simulink model "gm_interleaver_model"  (R2020b)
settings: Solver=FixedStepDiscrete  StartTime=0.0  StopTime=30  RelTol=1e-3
libraries: commrandsrc3 x1, hdlsllib x1
settings Model: Creator=wardo  LastModifiedBy=EFlores
settings DataIOCC: LimitDataPoints=on  SaveOutput=off  SaveTime=off
settings OptimizationCC: BlockReduction=off  ConditionallyExecuteInputs=off  DefaultParameterBehavior=Inlined  LifeSpan=inf
settings DebuggingCC: AlgebraicLoopMsg=error  InheritedTsInSrcMsg=none  SingleTaskRateTransMsg=error  AllowSymbolicDim=off  StrictBusMsg=ErrorOnBusTreatedAsVector  SFUnexpectedBacktrackingDiag=warning  SFNoUnconditionalDefaultTransitionDiag=warning  SFExecutionAtInitializationDiag=none  ArithmeticOperatorsInVariantConditions=warning
settings HardwareCC: ProdBitPerPointer=32  ProdBitPerSizeT=32  ProdBitPerPtrDiffT=32  ProdLargestAtomicFloat=None  ProdIntDivRoundTo=Undefined  ProdEndianess=Unspecified  ProdWordSize=32  ProdHWDeviceType=ASIC/FPGA->ASIC/FPGA  ProdEqTarget=off
settings SFSimCC: SimUseLocalCustomCode=off  CustomCodeUndefinedFunction=UseInterfaceOnly
settings RTWCC: RTWUseLocalCustomCode=off
settings CodeAppCC: StateflowObjectComments=on
settings GRTTargetCC: TargetLangStandard=C89/C90 (ANSI)
settings ConfigComp: CovScope=ReferencedModels  CovMetricSettings=dw  CovSaveCumulativeToWorkspaceVar=on  CovSaveSingleToWorkspaceVar=on  CovExternalEMLEnable=off  CovSFcnEnable=off

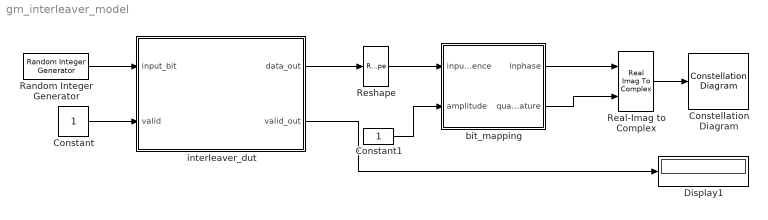
== system gm_interleaver_model ==
  Constant : Constant  OutDataTypeStr=boolean  SampleTime=-1
  Constant1 : Constant  OutMin=0  OutMax=5  OutDataTypeStr=fixdt(1,16)  SampleTime=-1
  Constellation Diagram : ConstellationDiagram
  Display1 : Display
  Random Integer Generator : commrandsrc3/Random Integer Generator  SetSize=2  SeedSource=Auto  Seed=0  SampleTime=1  SamplesPerFrame=1  OutputDataType=boolean  SimulateUsing=Interpreted execution
  Real-Imag to Complex : RealImagToComplex
  Reshape : Reshape
  bit_mapping : Subsystem
  interleaver_dut : Subsystem
  wires:
  Reshape/1 -> bit_mapping/1(input_sequence)
  Constant1/1 -> bit_mapping/2(amplitude)
  bit_mapping/2(quadrature) -> Real-Imag to Complex/2
  bit_mapping/1(inphase) -> Real-Imag to Complex/1
  Real-Imag to Complex/1 -> Constellation Diagram/1
  interleaver_dut/1(data_out) -> Reshape/1
  interleaver_dut/2(valid_out) -> Display1/1
  Constant/1 -> interleaver_dut/2(valid)
  Random Integer Generator/1 -> interleaver_dut/1(input_bit)

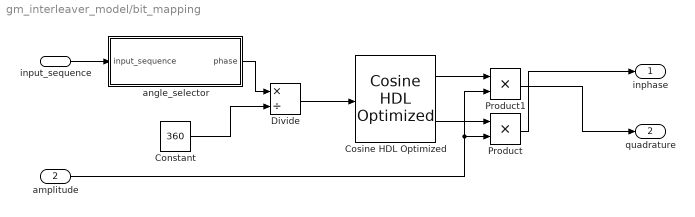
== system gm_interleaver_model/bit_mapping ==
  input_sequence : Inport
  amplitude : Inport  Port=2
  Constant : Constant  Value=360  OutDataTypeStr=fixdt(0,9,0)  SampleTime=-1
  Cosine HDL Optimized : hdlsllib/Lookup Tables/Cosine HDL Optimized  OutputFormula=sin(2*pi*u) and cos(2*pi*u)  NumDataPoints=32  TableDataTypeStr=fixdt(1,16,15)  SimulateLUTROMDelay=off
      settings: SourceProductBaseCode=SL
  Divide : Product  Inputs=*/  OutMin=0  OutMax=1  OutDataTypeStr=fixdt(1,16,14)  RndMeth=Zero  SaturateOnIntegerOverflow=on
  Product : Product
  Product1 : Product
  angle_selector : MATLAB Function  TreatAsAtomicUnit=on
  inphase : Outport  VectorParamsAs1DForOutWhenUnconnected=off
  quadrature : Outport  Port=2  VectorParamsAs1DForOutWhenUnconnected=off
  wires:
  Constant/1 -> Divide/2
  angle_selector/1(phase) -> Divide/1
  Divide/1 -> Cosine HDL Optimized/1
  Cosine HDL Optimized/1 -> Product1/1
  Cosine HDL Optimized/2 -> Product/1
  amplitude/1 -> Product/2, Product1/2
  input_sequence/1 -> angle_selector/1(input_sequence)
  Product1/1 -> quadrature/1
  Product/1 -> inphase/1

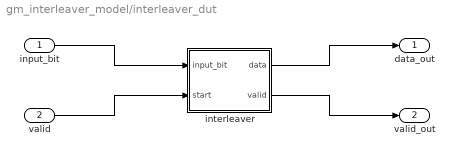
== system gm_interleaver_model/interleaver_dut ==
  input_bit : Inport  OutDataTypeStr=boolean  PortDimensions=1  SampleTime=1
  valid : Inport  Port=2  OutDataTypeStr=boolean  PortDimensions=1  SampleTime=1
  interleaver : Subsystem
  data_out : Outport  VectorParamsAs1DForOutWhenUnconnected=off
  valid_out : Outport  Port=2  VectorParamsAs1DForOutWhenUnconnected=off
  wires:
  input_bit/1 -> interleaver/1(input_bit)
  valid/1 -> interleaver/2(start)
  interleaver/1(data) -> data_out/1
  interleaver/2(valid) -> valid_out/1

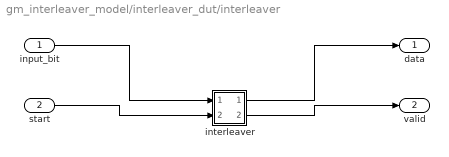
== system gm_interleaver_model/interleaver_dut/interleaver ==
  input_bit : Inport  OutDataTypeStr=boolean  PortDimensions=1  SampleTime=1
  start : Inport  Port=2  OutDataTypeStr=boolean  PortDimensions=1  SampleTime=1
  interleaver : MATLAB Function  TreatAsAtomicUnit=on
  data : Outport  VectorParamsAs1DForOutWhenUnconnected=off
  valid : Outport  Port=2
  wires:
  input_bit/1 -> interleaver/1(input_bit)
  start/1 -> interleaver/2(start)
  interleaver/1(data) -> data/1
  interleaver/2(valid) -> valid/1

== matlab function gm_interleaver_model/interleaver_dut/interleaver/interleaver ==
  settings: fimath=fimath('RoundingMethod', 'Floor','OverflowAction', 'Wrap','ProductMode', 'FullPrecision', 'SumMode', 'FullPrecision')
  data: input_bit input; data output; start input; valid output
function [data, valid] = fsm_interleaver(input_bit, start)
%#codegen

rows           = 21600;
columns        = 3;
state_iddle    = 0;
state_writting = 1;
state_reading  = 2;

persistent moore_state_reg;
if isempty(moore_state_reg)
    moore_state_reg = fi(0, 0, 2, 0);   
end

persistent counter;
if isempty(counter)
    counter = fi(1, 0, 16, 0);
end

persistent column;
if isempty(column)
    column = fi(1, 0, 8, 0);   
end

persistent buffer;
if isempty(buffer)
    buffer = fi(zeros(rows, columns), 0, 1, 0);
end

switch (moore_state_reg)
    
    case state_iddle
        counter = fi(1, 0, 16, 0);   
        column  = fi(1, 0, 8, 0);   
        buffer  = fi(zeros(rows, columns), 0, 1, 0);
        valid   = false;
        data    = fi([0 0 0], 0, 1, 0);
        if (~start)
            moore_state_reg(1) = state_iddle;
        else
            moore_state_reg(1) = state_writting;
            % Write first bit at the first position as it is the MSB
            buffer(counter, column) = input_bit;
            counter = fi(counter + 1, 0, 16, 0);
        end
        
    case state_writting
        buffer(counter, column) = input_bit;
        counter = fi(counter + 1, 0, 16, 0);
        if counter > rows
            counter = fi(1, 0, 16, 0);
            column  = fi(column + 1, 0, 8, 0);
            if (column > columns)
                moore_state_reg(1) = state_reading;
                counter = fi(1, 0, 16, 0);   
                column  = fi(1, 0, 8, 0);   
                valid   = true;
                data    = buffer(counter, :);
                counter = fi(counter + 1, 0, 16, 0);
            else
                data    = fi([0 0 0], 0, 1, 0);
                valid   = false;
            end
        else
            valid   = false;
            data    = fi([0 0 0], 0, 1, 0);
        end
    case state_reading
        data = buffer(counter, :);
        counter = fi(counter + 1, 0, 16, 0);
        if counter > rows
            moore_state_reg(1) = state_iddle;
        end
        valid = true;
    otherwise
        valid = false;
        data  = fi([0 0 0], 0, 1, 0);      
end

== matlab function gm_interleaver_model/bit_mapping/angle_selector ==
  settings: fimath=fimath('RoundingMethod', 'Floor','OverflowAction', 'Wrap','ProductMode', 'FullPrecision', 'SumMode', 'FullPrecision')
  data: input_sequence input; phase output
function phase = phase_selector(input_sequence)
%#codegen
% Receives a bit sequence and returns the angle in radians of the
% corresponding 8-psk constellation symbol. Gray encoding is used as stated
% in the DVB-S2 standard.
    tmp = 0; % Start at phase 0
    if(input_sequence(1)==0 && input_sequence(2)==0 && input_sequence(3)==1)
        tmp=0;
    elseif(input_sequence(1)==0 && input_sequence(2)==0 && input_sequence(3)==0)
        tmp=45;
    elseif(input_sequence(1)==1 && input_sequence(2)==0 && input_sequence(3)==0)
        tmp=90;
    elseif(input_sequence(1)==1 && input_sequence(2)==1 && input_sequence(3)==0)
        tmp=135;
    elseif(input_sequence(1)==0 && input_sequence(2)==1 && input_sequence(3)==0)
        tmp=180;
    elseif(input_sequence(1)==0 && input_sequence(2)==1 && input_sequence(3)==1)
        tmp=225;
    elseif(input_sequence(1)==1 && input_sequence(2)==1 && input_sequence(3)==1)
        tmp=270;
    elseif(input_sequence(1)==1 && input_sequence(2)==0 && input_sequence(3)==1)
        tmp=315;
    end
    % 9 bits necessary to represent 360 degrees.
    phase = fi(tmp, 0, 23, 14, hdlfimath);
